simulink model "cos_bank_2"  (Simulink 7.8)
settings: Solver=ode45  StartTime=0.0  StopTime=1-1e-3  RelTol=1e-3
values from neighbouring files (symbols this model uses):
  N = 2    [CFIR_1.m]    (also in TP_fdesign2.m = 128; cic_dezim1.m = ',num2str(N),')']); cic_dezim1_.m = ', num2str(N),' Gain = ',num2str(Hm.gain)]); cic_dezim2.m = ',num2str(N),')']))
  Ts = 1/fs    (= 6.25e-05)    [G722_1.m]    (also in adaptiv_2.m = 0.001; adaptiv_3.m = 0.001; adaptiv_4.m = 0.001; adaptiv_5.m = 0.001)
undefined symbols (not defined in the file or in its folder): hi, hit, magnitude
libraries: dspsigops x3, dspobslib x3, dspstat3 x2, dspbuff3 x1
settings Model: Creator=svenhoffmann  LastModifiedBy=josef  ExtModeAutoUpdateStatusClock=off
settings DataIOCC: SignalLoggingName=sigsOut
settings OptimizationCC: InitFltsAndDblsToZero=on
settings DebuggingCC: SaveWithParameterizedLinksMsg=none  SignalResolutionControl=TryResolveAllWithWarning  SolverPrmCheckMsg=none  MultiTaskDSMMsg=warning  MultiTaskCondExecSysMsg=none  FcnCallInpInsideContextMsg=Use local settings  StrictBusMsg=None
settings HardwareCC: TargetUnknown=on
settings RTWCC: IncludeERTFirstTime=on
settings GRTTargetCC: TargetFcnLib=ansi_tfl_tmw.mat

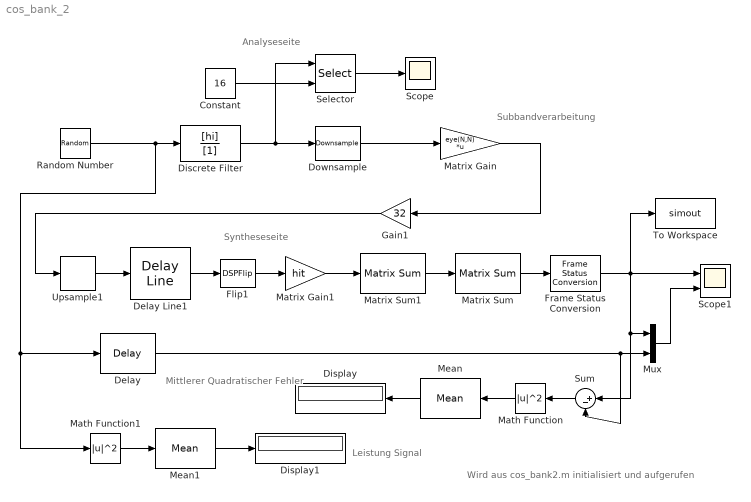
== system cos_bank_2 ==
  note: Subbandverarbeitung
  note: Analyseseite
  note: Syntheseseite
  note: Mittlerer Quadratischer
      |  Fehler
  note: Leistung Signal
  note: Wird aus cos_bank2.m initialisiert und aufgerufen
  Constant : Constant  Value=16
  Delay : dspsigops/Delay  InputProcessing=Inherited (this choice will be removed - see release notes)  dly_unit=Samples  delay=L  ic_detail=off  dif_ic_for_ch=off  dif_ic_for_dly=off  ic=0  reset_popup=None
  Delay Line1 : dspbuff3/Delay Line  siz=L  ic=0  directfeed=off  enable_output=off  hold_output=off  TreatMby1Signals=M channels (this choice will be removed - see release notes)
  Discrete Filter : DiscreteFilter  Numerator=[hi]  Denominator=[1]  SampleTime=Ts
  Display : Display
  Display1 : Display
  Downsample : dspsigops/Downsample  N=N  phase=0  InputProcessing=Inherited (this choice will be removed - see release notes)  RateOptions=Enforce single-rate processing  smode=Allow multirate  fmode=Maintain input frame size  ic=0
  Flip1 : DSPFlip
  Frame Status Conversion : dspobslib/Frame Status Conversion  growRefPort=off  outframe=Sample-based
  Gain1 : Gain  Gain=32  SaturateOnIntegerOverflow=on  OutDataTypeStr=Inherit: Same as input  ParamDataTypeStr=Inherit: Same as input
  Math Function : Math  Operator=magnitude^2  SaturateOnIntegerOverflow=on
  Math Function1 : Math  Operator=magnitude^2  SaturateOnIntegerOverflow=on
  Matrix Gain : Gain  Gain=eye(N,N)  Multiplication=Matrix(K*u)  SaturateOnIntegerOverflow=on  OutDataTypeStr=Inherit: Same as input  ParamDataTypeStr=Inherit: Same as input
  Matrix Gain1 : Gain  Gain=hit  SaturateOnIntegerOverflow=on  OutDataTypeStr=Inherit: Same as input  ParamDataTypeStr=Inherit: Same as input
  Matrix Sum : dspobslib/Matrix Sum  Dim=Rows  roundingMode=Floor  overflowMode=off
  Matrix Sum1 : dspobslib/Matrix Sum  Dim=Columns  roundingMode=Floor  overflowMode=off
  Mean : dspstat3/Mean  run=on  reset_popup=None  InputProcessing=Inherited (this choice will be removed - see release notes)  directionMode=Each column  dimension=1  treatSBRowAsCol=on  roiEnable=off  roiType=Rectangles  roiPortion=Entire ROI  roiOutput=Individual statistics for each ROI  roiFlag=off  outputDataTypeStr=Inherit: Same as accumulator  outputLastDataTypeStr=Inherit: Same as accumulator  outputMin=[]  outputMax=[]  roundingMode=Floor  overflowMode=off
  Mean1 : dspstat3/Mean  run=on  reset_popup=None  InputProcessing=Inherited (this choice will be removed - see release notes)  directionMode=Each column  dimension=1  treatSBRowAsCol=on  roiEnable=off  roiType=Rectangles  roiPortion=Entire ROI  roiOutput=Individual statistics for each ROI  roiFlag=off  outputDataTypeStr=Inherit: Same as accumulator  outputLastDataTypeStr=Inherit: Same as accumulator  outputMin=[]  outputMax=[]  roundingMode=Floor  overflowMode=off
  Mux : Mux  Inputs=2
  Random Number : RandomNumber  SampleTime=Ts
  Scope : Scope
      settings: YMin=-0.0125  YMax=0.0125
  Scope1 : Scope  NumInputPorts=2
      settings: TimeRange=0.2  YMin=-2.25~-2.25  YMax=2.75~2.75
  Selector : Selector  InputPortWidth=N  IndexOptions=Index vector (port)  Indices=[1 3]  OutputSizes=1
  Sum : Sum  Inputs=|+-  SaturateOnIntegerOverflow=on
  To Workspace : ToWorkspace  VariableName=simout  SampleTime=-1  SaveFormat=Array
  Upsample1 : dspsigops/Upsample  N=N  phase=0  InputProcessing=Inherited (this choice will be removed - see release notes)  RateOptions=Allow multirate processing  ic=0  mode=Unused parameter value
  wires:
  Discrete Filter/1 -> Selector/1, Downsample/1
  Constant/1 -> Selector/2
  Selector/1 -> Scope/1
  Downsample/1 -> Matrix Gain/1
  Frame Status Conversion/1 -> Scope1/1, Mux/1, Sum/1, To Workspace/1
  Matrix Gain1/1 -> Matrix Sum1/1
  Matrix Sum/1 -> Frame Status Conversion/1
  Matrix Sum1/1 -> Matrix Sum/1
  Mux/1 -> Scope1/2
  Delay/1 -> Mux/2, Sum/2
  Sum/1 -> Math Function/1
  Mean/1 -> Display/1
  Math Function/1 -> Mean/1
  Upsample1/1 -> Delay Line1/1
  Delay Line1/1 -> Flip1/1
  Flip1/1 -> Matrix Gain1/1
  Matrix Gain/1 -> Gain1/1
  Gain1/1 -> Upsample1/1
  Math Function1/1 -> Mean1/1
  Mean1/1 -> Display1/1
  Random Number/1 -> Discrete Filter/1, Delay/1, Math Function1/1
